simulink model "reduced_model"  (R2015b)
settings: Solver=FixedStepAuto  StartTime=0.0  StopTime=30  FixedStep=Ts  MaxStep=0.005  RelTol=1e-3
InitFcn:
  | Ts=0.01;
values from neighbouring files (symbols this model uses):
  aa = Ti*A*T    [hsvdModel_2area.m]
  bb = Ti*B    [hsvdModel_2area.m]
  cc = C*Ti    [hsvdModel_2area.m]
  dPL1 = 1    [hsvdModel_2area.m]
  dPL2 = 0    [hsvdModel_2area.m]
undefined symbols (not defined in the file or in its folder): a, b, c, T
settings Model: Creator=Majidi  LastModifiedBy=Admin
settings DataIOCC: SaveFormat=Array
settings OptimizationCC: ExpressionDepthLimit=2147483647
settings DebuggingCC: UnderspecifiedInitializationDetection=Classic  MergeDetectMultiDrivingBlocksExec=none  SolverPrmCheckMsg=warning  StateNameClashWarn=warning
settings HardwareCC: ProdBitPerPointer=32  ProdLargestAtomicFloat=None  ProdIntDivRoundTo=Undefined  ProdEndianess=Unspecified  ProdWordSize=32  ProdHWDeviceType=32-bit Generic
settings GRTTargetCC: GeneratePreprocessorConditionals=Disable all
settings ConfigComp: CovModelRefEnable=Off

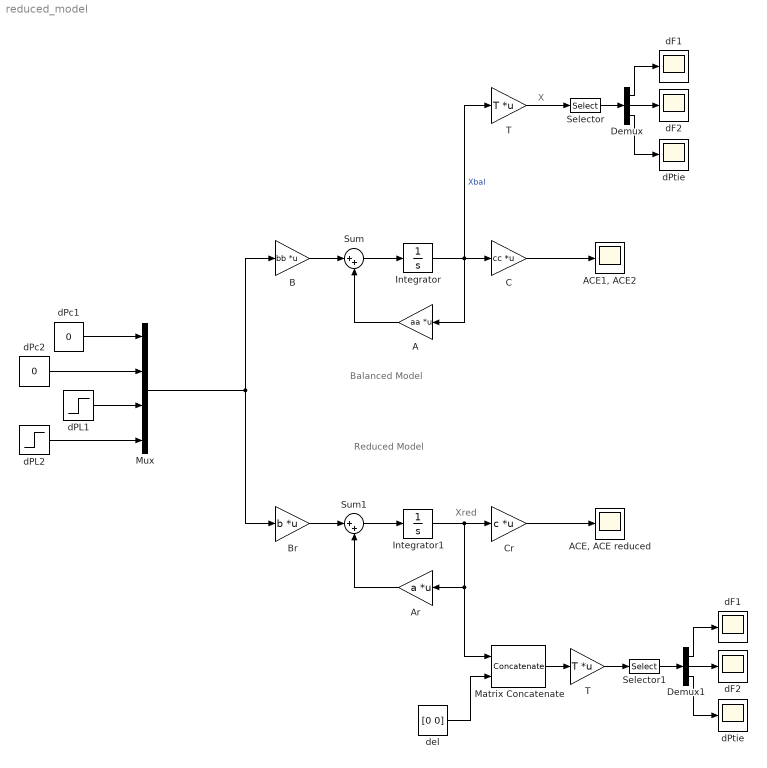
== system reduced_model ==
  note: Reduced Model
  note: Balanced Model
  note: X
  note: Xred
  A : Gain  Gain=aa  Multiplication=Matrix(K*u)
  "ACE, ACE reduced" : Scope
  "ACE1, ACE2" : Scope
  Ar : Gain  Gain=a  Multiplication=Matrix(K*u)
  B : Gain  Gain=bb  Multiplication=Matrix(K*u)
  Br : Gain  Gain=b  Multiplication=Matrix(K*u)
  C : Gain  Gain=cc  Multiplication=Matrix(K*u)
  Cr : Gain  Gain=c  Multiplication=Matrix(K*u)
  Demux : Demux  Outputs=3
  Demux1 : Demux  Outputs=3
  Integrator : Integrator
  Integrator1 : Integrator
  Matrix Concatenate : Concatenate  ConcatenateDimension=2
  Mux : Mux
  Selector : Selector  InputPortWidth=7  IndexOptions=Index vector (dialog)  Indices=[3 4 7]  OutputSizes=1
  Selector1 : Selector  InputPortWidth=7  IndexOptions=Index vector (dialog)  Indices=[3 4 7]  OutputSizes=1
  Sum : Sum  Inputs=|++
  Sum1 : Sum  Inputs=|++
  T : Gain  Gain=T  Multiplication=Matrix(K*u)
  "T " : Gain  Gain=T  Multiplication=Matrix(K*u)
  dF1 : Scope
  "dF1 " : Scope
  dF2 : Scope
  "dF2 " : Scope
  dPL1 : Step  After=dPL1  SampleTime=0
  dPL2 : Step  After=dPL2  SampleTime=0
  dPc1 : Constant  Value=0
  dPc2 : Constant  Value=0
  dPtie : Scope
  "dPtie " : Scope
  del : Constant  Value=[0 0]
  wires:
  B/1 -> Sum/1
  Sum/1 -> Integrator/1
  A/1 -> Sum/2
  Integrator/1 -> T/1, A/1, C/1  "Xbal"
  C/1 -> "ACE1, ACE2"/1
  dPL1/1 -> Mux/3
  dPL2/1 -> Mux/4
  dPc1/1 -> Mux/1
  dPc2/1 -> Mux/2
  Demux/1 -> dF1/1
  Demux/2 -> dF2/1
  Demux/3 -> dPtie/1
  Selector/1 -> Demux/1
  Br/1 -> Sum1/1
  Sum1/1 -> Integrator1/1
  Ar/1 -> Sum1/2
  Integrator1/1 -> Cr/1, Ar/1, Matrix Concatenate/1
  Mux/1 -> B/1, Br/1
  T/1 -> Selector/1
  Cr/1 -> "ACE, ACE reduced"/1
  del/1 -> Matrix Concatenate/2
  Matrix Concatenate/1 -> "T "/1
  "T "/1 -> Selector1/1
  Demux1/1 -> "dF1 "/1
  Demux1/2 -> "dF2 "/1
  Demux1/3 -> "dPtie "/1
  Selector1/1 -> Demux1/1
